simulink model "esercizio_1_massaMollaSmorzatore"  (R2024a)
settings: Solver=VariableStepAuto  StartTime=0.0  StopTime=10  RelTol=1e-3
PreLoadFcn:
  | % --------------------
  | % system's parameters:
  | % --------------------
  | 
  | M = 50 % massa
  | K = 0.02 % costante elastica
  | S = 0.02 % costante smorzatore
  | 
  | % --------------------
  | % desired eigenvalues
  | % --------------------
  | 
  | eig_G = 1*[-1 -2 ]
  | 
  | % --------------------
  | % matrix and initial conditions
  | % --------------------
  | 
  | A = [   0     1    ;
  |       -K/M  -S/M   ]
  | 
  | 
  | B = [  0  ;
  |       1/M ]
  | 
  | 
  | C = [ 1 0 ;
  |       0 1 ]
  | 
  | D = zeros(size(C,1),size(B,2))
  | 
  | 
  | dimx = size(A,1)  % quindi dimx = 2
  | dimu = size(B,2)  % quindi dimu = 1
  | dimy = size(C,1)  % quindi dimy = 2
  | 
  | x0 = [20; % posizione iniziale
  |       100] % velocità iniziale
  | 
  | % --------------------
  | % certainty-equivalence state-feedback controller
  | % --------------------
  | 
  | G = place(A,B,eig_G) % costruisce matrice G dati gli autovalori desiderati
libraries: vrlib x2, sldrtlib x1
settings Model: Creator=39342  LastModifiedBy=simone

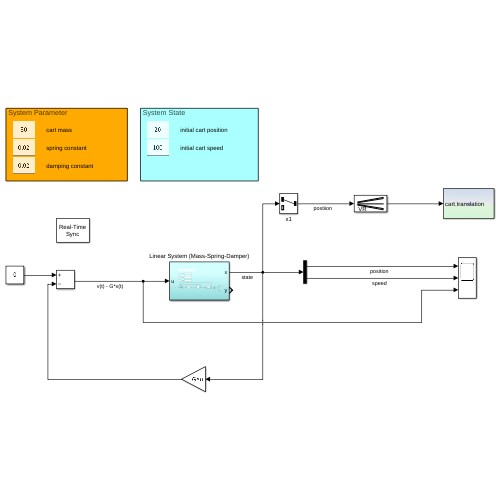
[thumbnail: Simulink's stored preview of the top-level diagram]
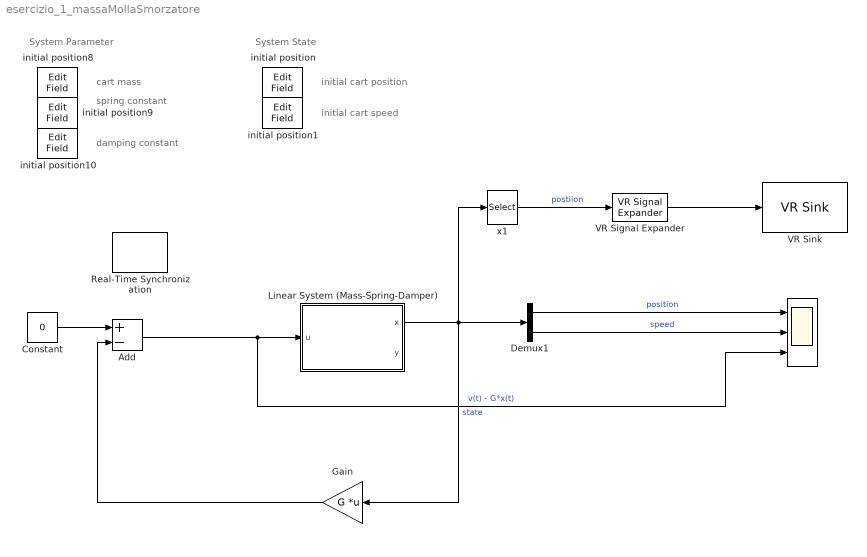
== system esercizio_1_massaMollaSmorzatore ==
  note: cart mass
  note: initial cart speed
  note: System State
  note: System Parameter
  note: spring constant
  note: initial cart position
  note: damping constant
  " " : Scope  NumInputPorts=3
  Add : Sum  Inputs=+-
  Constant : Constant  Value=0
  Demux1 : Demux  Outputs=2
  Gain : Gain  Gain=G  Multiplication=Matrix(K*u)
  Linear System (Mass-Spring-Damper) : Subsystem
  Real-Time Synchronization : sldrtlib/Real-Time Synchronization  SampleTime=0.01  MaxMissedTicks=100  ShowMissedTicks=off  YieldWhenWaiting=off
  VR Signal Expander : vrlib/VR Signal Expander  outwidth=3  outidx=[1]
  VR Sink : vrlib/VR Sink  InstantiateOnLoad=on  SampleTime=0.1  ViewEnable=on  RemoteChange=off  RemoteView=off  FieldsWritten=cart.translation.3.1.1.double  WorldFileName=animazioneCarrello.x3d  AutoView=on  VideoDimensions=[]  AllowVariableSize=off
  initial position{,1,8..10} (5 alike) : EditField  LabelPosition=Hide  ShowInitialText=on  Alignment=Center
  x1 : Selector  InputPortWidth=2  IndexOptions=Index vector (dialog)  Indices=[1]  OutputSizes=1
  wires:
  Gain/1 -> Add/2
  Constant/1 -> Add/1
  Add/1 -> Linear System (Mass-Spring-Damper)/1(u), " "/3  "v(t) - G*x(t)"
  Linear System (Mass-Spring-Damper)/1(x) -> x1/1, Demux1/1, Gain/1  "state"
  Demux1/2 -> " "/2  "speed"
  Demux1/1 -> " "/1  "position"
  x1/1 -> VR Signal Expander/1  "postiion"
  VR Signal Expander/1 -> VR Sink/1

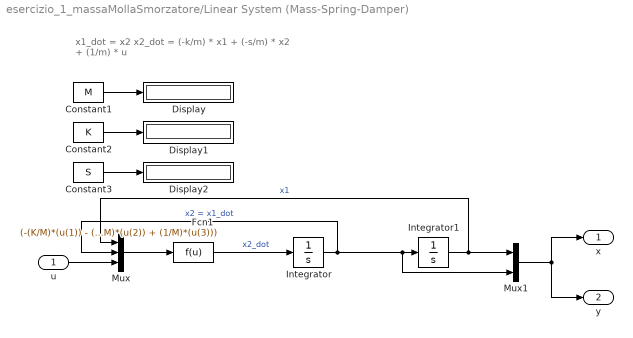
== system esercizio_1_massaMollaSmorzatore/Linear System (Mass-Spring-Damper) ==
  note: x1_dot = x2
      | x2_dot = (-k/m) * x1 + (-s/m) * x2 + (1/m) * u
  u : Inport
  Constant1 : Constant  Value=M
  Constant2 : Constant  Value=K
  Constant3 : Constant  Value=S
  Display : Display
  Display1 : Display
  Display2 : Display
  Fcn1 : Fcn  Expr=(-(K/M)*(u(1)) - (S/M)*(u(2)) + (1/M)*(u(3)))
  Integrator : Integrator  InitialCondition=x0(2)
  Integrator1 : Integrator  InitialCondition=x0(1)
  Mux : Mux  Inputs=3
  Mux1 : Mux  Inputs=2
  x : Outport
  y : Outport  Port=2
  wires:
  Fcn1/1 -> Integrator/1  "x2_dot"
  Integrator/1 -> Mux/2, Mux1/2, Integrator1/1  "x2 = x1_dot"
  Mux/1 -> Fcn1/1
  u/1 -> Mux/3
  Integrator1/1 -> Mux/1, Mux1/1  "x1"
  Mux1/1 -> x/1, y/1
  Constant2/1 -> Display1/1
  Constant3/1 -> Display2/1
  Constant1/1 -> Display/1
